simulink model "AutoLIB"  (R2015a)
settings: Solver=FixedStepDiscrete  StartTime=0.0  StopTime=10  FixedStep=0.01  RelTol=1e-3
undefined symbols (not defined in the file or in its folder): sigbuilder_block
settings Model: ModifiedByFormat=Unknown  NumberOfSteps=10  Creator=Unknown  LastModifiedBy=Unknown
settings OptimizationCC: OptimizeModelRefInitCode=on  LifeSpan=1
settings RTWCC: SystemTargetFile=ert.tlc  TemplateMakefile=ert_default_tmf  Description=Embedded Coder
settings CodeAppCC: IgnoreCustomStorageClasses=off
settings ERTTargetCC: ParMdlRefBuildCompliant=on  CompOptLevelCompliant=on  ConcurrentExecutionCompliant=on  ERTFirstTimeCompliant=on  SupportContinuousTime=off  SupportVariableSizeSignals=off  ModelStepFunctionPrototypeControlCompliant=on  CPPClassGenCompliant=on  InlinedParameterPlacement=Hierarchical  ERTCustomFileTemplate=example_file_process.tlc
settings ConfigComp: Description=Design Verifier Custom Configuration Component  DVMaxTestCaseSteps=500  DVTestSuiteOptimization=CombinedObjectives (Nonlinear Extended)

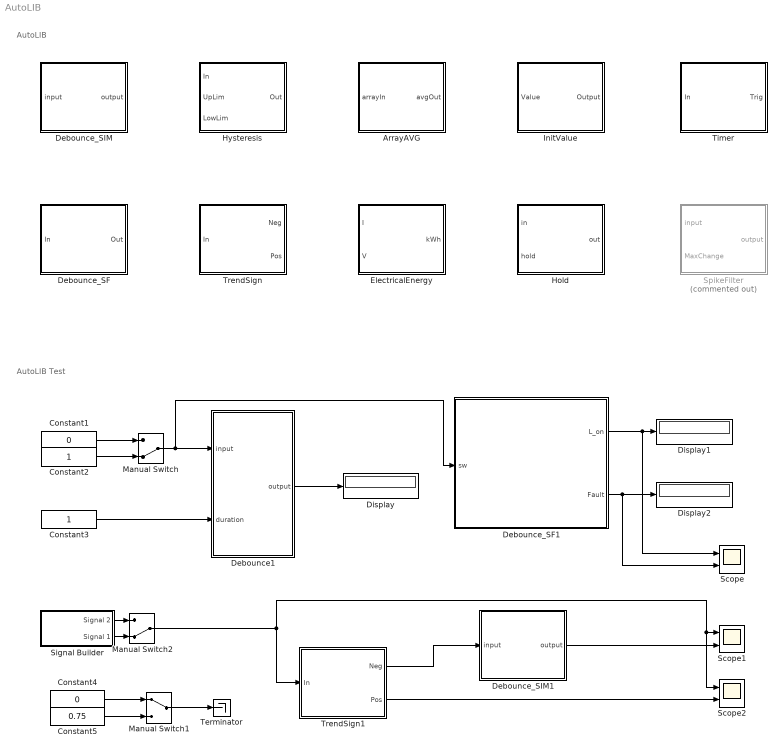
== system AutoLIB ==
  note: AutoLIB
  note: AutoLIB Test
  ArrayAVG : Subsystem  TreatAsAtomicUnit=on
      mask Display:
      | port_label('input',1,'arrIn')
      | port_label('output',1,'avgOut')
      | 
      | 
      | plot([0.30, 0.75],[0.25, 0.25])
      | plot([0.30, 0.30],[0.25, 0.75])
      | 
      | plot([0.55, 0.70],[0.40, 0.40])
      | 
      | color('red');
      | plot([0.30, 0.50],[0.50, 0.50])
      | 
      | color('blue');
      | plot([0.30, 0.50],[0.30, 0.30])
      | 
      | color('green');
      | plot([0.30, 0.50],[0.40, 0.40])
  Constant1 : Constant  Value=0  OutDataTypeStr=boolean
  Constant2 : Constant  OutDataTypeStr=boolean
  Constant3 : Constant  OutDataTypeStr=boolean
  Constant4 : Constant  Value=0  OutDataTypeStr=double
  Constant5 : Constant  Value=0.75  OutDataTypeStr=double
  Debounce1 : Subsystem
  Debounce_SF : Subsystem  TreatAsAtomicUnit=on  mask{Duration=0}
      mask Display:
      | port_label('input',1,'In')
      | port_label('output',1,'Out')
      | 
      | disp(['Debounce: ' num2str(double(Duration)) '\n\n\n\n\n'])
      | 
      | plot([0.30, 0.75],[0.25, 0.25])
      | plot([0.30, 0.30],[0.25, 0.75])
      | 
      | plot([0.30, 0.32],[0.50, 0.50])
      | plot([0.32, 0.32],[0.50, 0.25])
      | plot([0.32, 0.34],[0.25, 0.25])
      | plot([0.34, 0.34],[0.25, 0.50])
      | 
      | plot([0.34, 0.36],[0.50, 0.50])
      | plot([0.36, 0.36],[0.50, 0.25])
      | plot([0.36, 0.38],[0.25, 0.25])
      | plot([0.38, 0.38],[0.25, 0.50])
      | plot([0.38, 0.42],[0.50, 0.50])
      | 
      | color('red');
      | plot([0.42, 0.42],[0.25, 0.50])
      | plot([0.42, 0.52],[0.50, 0.50])
      | plot([0.52, 0.52],[0.50, 0.25])
      | plot([0.52, 0.52],[0.25, 0.25])
  Debounce_SF1 : Stateflow chart  TreatAsAtomicUnit=on
  Debounce_SIM : Subsystem  TreatAsAtomicUnit=on  mask{Duration=3}
      mask prompts: Duration "Debounce Duration"
      mask help: The bouncing action can produce transient signals that do not represent a true change of state, Debounce block avoids these bouncing state.
      mask Display:
      | port_label('input',1,'In')
      | port_label('output',1,'Out')
      | 
      | disp(['Debounce: ' num2str(double(Duration)) '\n\n\n\n\n'])
      | 
      | plot([0.30, 0.75],[0.25, 0.25])
      | plot([0.30, 0.30],[0.25, 0.75])
      | 
      | plot([0.30, 0.32],[0.50, 0.50])
      | plot([0.32, 0.32],[0.50, 0.25])
      | plot([0.32, 0.34],[0.25, 0.25])
      | plot([0.34, 0.34],[0.25, 0.50])
      | 
      | plot([0.34, 0.36],[0.50, 0.50])
      | plot([0.36, 0.36],[0.50, 0.25])
      | plot([0.36, 0.38],[0.25, 0.25])
      | plot([0.38, 0.38],[0.25, 0.50])
      | plot([0.38, 0.42],[0.50, 0.50])
      | 
      | color('red');
      | plot([0.42, 0.42],[0.25, 0.50])
      | plot([0.42, 0.52],[0.50, 0.50])
      | plot([0.52, 0.52],[0.50, 0.25])
      | plot([0.52, 0.52],[0.25, 0.25])
  Debounce_SIM1 : Subsystem  mask{Duration=2}
      mask prompts: Duration "Debounce Duration"
      mask help: The bouncing action can produce transient signals that do not represent a true change of state, Debounce block avoids these bouncing state.
      mask Display:
      | port_label('input',1,'In')
      | port_label('output',1,'Out')
      | 
      | disp(['Debounce: ' num2str(double(Duration)) '\n\n\n\n\n'])
      | 
      | plot([0.30, 0.75],[0.25, 0.25])
      | plot([0.30, 0.30],[0.25, 0.75])
      | 
      | plot([0.30, 0.32],[0.50, 0.50])
      | plot([0.32, 0.32],[0.50, 0.25])
      | plot([0.32, 0.34],[0.25, 0.25])
      | plot([0.34, 0.34],[0.25, 0.50])
      | 
      | plot([0.34, 0.36],[0.50, 0.50])
      | plot([0.36, 0.36],[0.50, 0.25])
      | plot([0.36, 0.38],[0.25, 0.25])
      | plot([0.38, 0.38],[0.25, 0.50])
      | plot([0.38, 0.42],[0.50, 0.50])
      | 
      | color('red');
      | plot([0.42, 0.42],[0.25, 0.50])
      | plot([0.42, 0.52],[0.50, 0.50])
      | plot([0.52, 0.52],[0.50, 0.25])
      | plot([0.52, 0.52],[0.25, 0.25])
  Display : Display
  Display1 : Display
  Display2 : Display
  ElectricalEnergy : Subsystem  TreatAsAtomicUnit=on  mask{SampleTime=0}
      mask Display: plot([10 20 30 40], [10 20 10 15])
  Hold : Subsystem  TreatAsAtomicUnit=on  mask{StepTime=0.01}
      mask prompts: StepTime "Sample Time"
      mask help: Output is fixed at TRUE for HOLD TIME after falling edge of Input.
      mask Display:
      | port_label('input',1,'In')
      | port_label('input',2,'Hold')
      | port_label('output',1,'Out')
      | 
      | plot([0.30, 0.75],[0.25, 0.25])
      | plot([0.30, 0.30],[0.25, 0.75])
      | plot([0.30, 0.60],[0.50, 0.50])
      | plot([0.60, 0.60],[0.50, 0.25])
  Hysteresis : Subsystem  TreatAsAtomicUnit=on
      mask Display:
      | plot([10 20 30 40], [10 20 10 15])
      | color('red');
      | plot([10 40], [17 17])
      | plot([10 40], [13 13])
  InitValue : Subsystem  TreatAsAtomicUnit=on  mask{InitValue=3, SampleTime=-1}
      mask Display:
      | disp(['Initial value: ' num2str(double(InitValue)) '\n\n\n\n'])
      | 
      | plot([0.30, 0.75],[0.25, 0.25])
      | plot([0.30, 0.30],[0.25, 0.75])
      | 
      | plot([0.30, 0.32],[0.50, 0.50])
      | plot([0.34, 0.36],[0.50, 0.50])
      | plot([0.38, 0.40],[0.50, 0.50])
      | plot([0.42, 0.44],[0.50, 0.50])
      | plot([0.46, 0.48],[0.50, 0.50])
      | 
      | plot([0.50, 0.60],[0.50, 0.50])
      | plot([0.60, 0.60],[0.50, 0.25])
  Manual Switch : ManualSwitch  CurrentSetting=0
  Manual Switch1 : ManualSwitch
  Manual Switch2 : ManualSwitch  CurrentSetting=0
  Scope : Scope  NumInputPorts=2
      settings: YMin=0~0  YMax=1~1
  Scope1 : Scope  NumInputPorts=2
      settings: YMin=-0.01~-1  YMax=-0.0092~1
  Scope2 : Scope  NumInputPorts=2
      settings: YMin=-0.01~-1  YMax=-0.0092~1  SaveName=ScopeData2
  Signal Builder : Subsystem  Tag=STV Subsys  LoadFcn=sigbuilder_block('load');  StartFcn=sigbuilder_block('start');  StopFcn=sigbuilder_block('stop');  ClipboardFcn=sigbuilder_block('clipboard');  mask(Sigbuilder block){}
      mask help: Simulink:masks:SigbuilderBlock_MD
      mask init:
      | if ~strcmp(get_param(bdroot(gcbh),'SimulationStatus'),'stopped') tuvar = sigbuilder_block('maskInit'); end
      settings: CopyFcn=sigbuilder_block('copy');  DeleteFcn=sigbuilder_block('delete');  ModelCloseFcn=sigbuilder_block('modelClose');  PreSaveFcn=sigbuilder_block('preSave');  PauseFcn=sigbuilder_block('pause');  ContinueFcn=sigbuilder_block('continue');  NameChangeFcn=sigbuilder_block('namechange');  OpenFcn=sigbuilder_block('open',[437.6 199.2 550.4 400 ]);  CloseFcn=sigbuilder_block('close');
      mask Display: plot(0, 0, 100, 100,[2, 2, 32, 32, 2], [68, 8, 8, 68, 68],[32, 2], [38, 38], [32, 19, 2],[53, 60, 44], [32, 17, 17, 2],[16, 16, 31, 31]);txt = getActiveGroup(gcbh);text(2, 100, txt,'verticalAlignment', 'top');
  SpikeFilter : Subsystem  Commented=on
  Terminator : Terminator
  Timer : Subsystem  TreatAsAtomicUnit=on  mask{Limit=3}
      mask Display:
      | disp(['Timer Target: ' num2str(double(Limit)) '\n\n\n\n'])
      | 
      | 
      | plot([0.30, 0.75],[0.30, 0.30])
      | plot([0.30, 0.30],[0.30, 0.70])
      | plot([0.30, 0.45],[0.30, 0.60])
      | 
      | 
      | color('red');
      | plot([0.45, 0.75],[0.60, 0.60])
  TrendSign : Subsystem  TreatAsAtomicUnit=on
      settings: MinAlgLoopOccurrences=on
      mask Display: fprintf('d/dt');
  TrendSign1 : Subsystem
      mask Display: fprintf('d/dt');
  wires:
  Manual Switch/1 -> Debounce1/1(input), Debounce_SF1/1(sw)
  Constant3/1 -> Debounce1/2(duration)
  Constant1/1 -> Manual Switch/1
  Debounce_SF1/1(L_on) -> Scope/1, Display1/1
  Debounce_SF1/2(Fault) -> Scope/2, Display2/1
  Debounce1/1(output) -> Display/1
  Constant2/1 -> Manual Switch/2
  Manual Switch1/1 -> Terminator/1
  Constant4/1 -> Manual Switch1/1
  Constant5/1 -> Manual Switch1/2
  Signal Builder/1(Signal 2) -> Manual Switch2/1
  Signal Builder/2(Signal 1) -> Manual Switch2/2
  Manual Switch2/1 -> TrendSign1/1(In), Scope2/1, Scope1/1
  Debounce_SIM1/1(output) -> Scope1/2
  TrendSign1/1(Neg) -> Debounce_SIM1/1(input)
  TrendSign1/2(Pos) -> Scope2/2

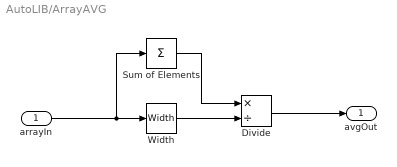
== system AutoLIB/ArrayAVG ==
  arrayIn : Inport
  Divide : Product  Inputs=*/
  Sum of Elements : Sum  Inputs=+
  Width : Width
  avgOut : Outport
  wires:
  Sum of Elements/1 -> Divide/1
  Width/1 -> Divide/2
  arrayIn/1 -> Width/1, Sum of Elements/1
  Divide/1 -> avgOut/1

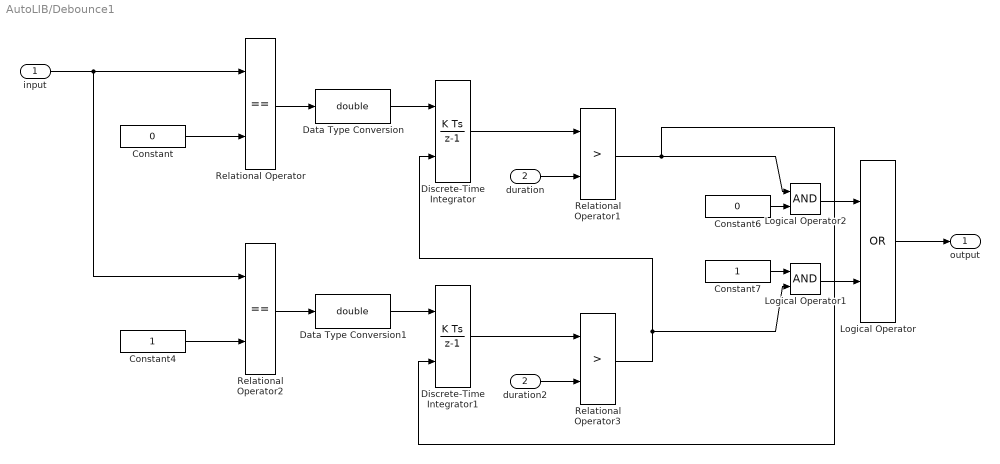
== system AutoLIB/Debounce1 ==
  input : Inport
  duration : Inport  Port=2
  Constant : Constant  Value=0  OutDataTypeStr=boolean
  Constant4 : Constant  OutDataTypeStr=boolean
  Constant6 : Constant  Value=0  OutDataTypeStr=boolean
  Constant7 : Constant  OutDataTypeStr=boolean
  Data Type Conversion : DataTypeConversion  OutDataTypeStr=double
  Data Type Conversion1 : DataTypeConversion  OutDataTypeStr=double
  Discrete-Time Integrator : DiscreteIntegrator  ExternalReset=rising  InitialConditionSetting=State (most efficient)  SampleTime=0.01
  Discrete-Time Integrator1 : DiscreteIntegrator  ExternalReset=rising  InitialConditionSetting=State (most efficient)  SampleTime=0.01
  Logical Operator : Logic  Operator=OR  AllPortsSameDT=off  OutDataTypeStr=boolean
  Logical Operator1 : Logic  AllPortsSameDT=off  OutDataTypeStr=boolean
  Logical Operator2 : Logic  AllPortsSameDT=off  OutDataTypeStr=boolean
  Relational Operator : RelationalOperator  Operator===  OutDataTypeStr=boolean
  Relational Operator1 : RelationalOperator  Operator=>  OutDataTypeStr=boolean
  Relational Operator2 : RelationalOperator  Operator===  OutDataTypeStr=boolean
  Relational Operator3 : RelationalOperator  Operator=>  OutDataTypeStr=boolean
  duration2 : InportShadow  Port=2
  output : Outport
  wires:
  Constant7/1 -> Logical Operator1/1
  Constant6/1 -> Logical Operator2/2
  Discrete-Time Integrator1/1 -> Relational Operator3/1
  Relational Operator3/1 -> Logical Operator1/2, Discrete-Time Integrator/2
  duration2/1 -> Relational Operator3/2
  input/1 -> Relational Operator/1, Relational Operator2/1
  Relational Operator2/1 -> Data Type Conversion1/1
  Data Type Conversion1/1 -> Discrete-Time Integrator1/1
  Constant4/1 -> Relational Operator2/2
  Data Type Conversion/1 -> Discrete-Time Integrator/1
  Logical Operator/1 -> output/1
  Logical Operator2/1 -> Logical Operator/1
  Logical Operator1/1 -> Logical Operator/2
  Relational Operator1/1 -> Logical Operator2/1, Discrete-Time Integrator1/2
  Relational Operator/1 -> Data Type Conversion/1
  Discrete-Time Integrator/1 -> Relational Operator1/1
  duration/1 -> Relational Operator1/2
  Constant/1 -> Relational Operator/2

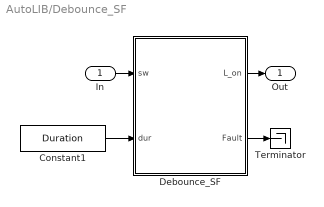
== system AutoLIB/Debounce_SF ==
  In : Inport
  Constant1 : Constant  Value=Duration  SampleTime=-1
  Debounce_SF : Stateflow chart  TreatAsAtomicUnit=on
  Terminator : Terminator
  Out : Outport
  wires:
  In/1 -> Debounce_SF/1(sw)
  Debounce_SF/1(L_on) -> Out/1
  Debounce_SF/2(Fault) -> Terminator/1
  Constant1/1 -> Debounce_SF/2(dur)

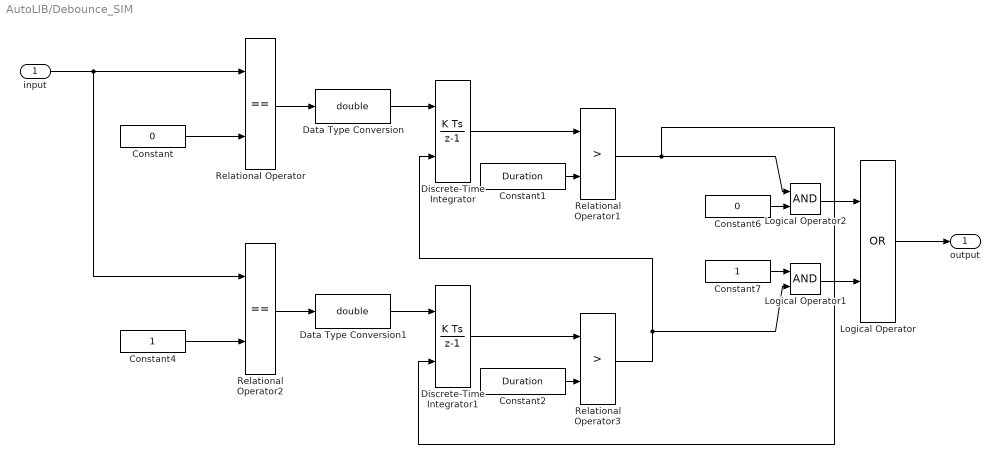
== system AutoLIB/Debounce_SIM ==
  input : Inport
  Constant : Constant  Value=0  OutDataTypeStr=boolean
  Constant1 : Constant  Value=Duration  SampleTime=-1
  Constant2 : Constant  Value=Duration  SampleTime=-1
  Constant4 : Constant  OutDataTypeStr=boolean
  Constant6 : Constant  Value=0  OutDataTypeStr=boolean
  Constant7 : Constant  OutDataTypeStr=boolean
  Data Type Conversion : DataTypeConversion  OutDataTypeStr=double
  Data Type Conversion1 : DataTypeConversion  OutDataTypeStr=double
  Discrete-Time Integrator : DiscreteIntegrator  ExternalReset=rising  InitialConditionSetting=State (most efficient)  SampleTime=0.01
  Discrete-Time Integrator1 : DiscreteIntegrator  ExternalReset=rising  InitialConditionSetting=State (most efficient)  SampleTime=0.01
  Logical Operator : Logic  Operator=OR  AllPortsSameDT=off  OutDataTypeStr=boolean
  Logical Operator1 : Logic  AllPortsSameDT=off  OutDataTypeStr=boolean
  Logical Operator2 : Logic  AllPortsSameDT=off  OutDataTypeStr=boolean
  Relational Operator : RelationalOperator  Operator===  OutDataTypeStr=boolean
  Relational Operator1 : RelationalOperator  Operator=>  OutDataTypeStr=boolean
  Relational Operator2 : RelationalOperator  Operator===  OutDataTypeStr=boolean
  Relational Operator3 : RelationalOperator  Operator=>  OutDataTypeStr=boolean
  output : Outport
  wires:
  Constant/1 -> Relational Operator/2
  Constant1/1 -> Relational Operator1/2
  Discrete-Time Integrator/1 -> Relational Operator1/1
  Relational Operator/1 -> Data Type Conversion/1
  Relational Operator1/1 -> Discrete-Time Integrator1/2, Logical Operator2/1
  Logical Operator1/1 -> Logical Operator/2
  Logical Operator2/1 -> Logical Operator/1
  Logical Operator/1 -> output/1
  Data Type Conversion/1 -> Discrete-Time Integrator/1
  Constant4/1 -> Relational Operator2/2
  Data Type Conversion1/1 -> Discrete-Time Integrator1/1
  Relational Operator2/1 -> Data Type Conversion1/1
  input/1 -> Relational Operator2/1, Relational Operator/1
  Relational Operator3/1 -> Discrete-Time Integrator/2, Logical Operator1/2
  Discrete-Time Integrator1/1 -> Relational Operator3/1
  Constant6/1 -> Logical Operator2/2
  Constant7/1 -> Logical Operator1/1
  Constant2/1 -> Relational Operator3/2

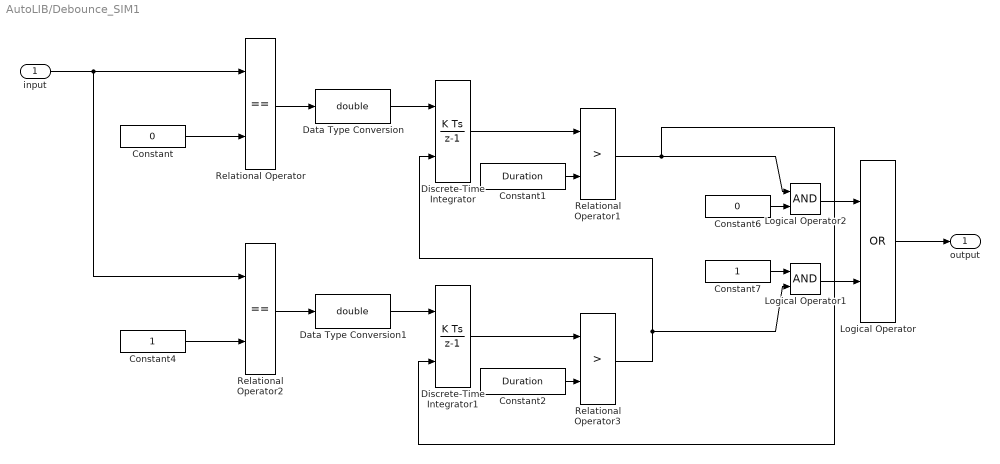
== system AutoLIB/Debounce_SIM1 ==
  input : Inport
  Constant : Constant  Value=0  OutDataTypeStr=boolean
  Constant1 : Constant  Value=Duration  SampleTime=-1
  Constant2 : Constant  Value=Duration  SampleTime=-1
  Constant4 : Constant  OutDataTypeStr=boolean
  Constant6 : Constant  Value=0  OutDataTypeStr=boolean
  Constant7 : Constant  OutDataTypeStr=boolean
  Data Type Conversion : DataTypeConversion  OutDataTypeStr=double
  Data Type Conversion1 : DataTypeConversion  OutDataTypeStr=double
  Discrete-Time Integrator : DiscreteIntegrator  ExternalReset=rising  InitialConditionSetting=State (most efficient)  SampleTime=0.01
  Discrete-Time Integrator1 : DiscreteIntegrator  ExternalReset=rising  InitialConditionSetting=State (most efficient)  SampleTime=0.01
  Logical Operator : Logic  Operator=OR  AllPortsSameDT=off  OutDataTypeStr=boolean
  Logical Operator1 : Logic  AllPortsSameDT=off  OutDataTypeStr=boolean
  Logical Operator2 : Logic  AllPortsSameDT=off  OutDataTypeStr=boolean
  Relational Operator : RelationalOperator  Operator===  OutDataTypeStr=boolean
  Relational Operator1 : RelationalOperator  Operator=>  OutDataTypeStr=boolean
  Relational Operator2 : RelationalOperator  Operator===  OutDataTypeStr=boolean
  Relational Operator3 : RelationalOperator  Operator=>  OutDataTypeStr=boolean
  output : Outport
  wires:
  Constant2/1 -> Relational Operator3/2
  Constant7/1 -> Logical Operator1/1
  Constant6/1 -> Logical Operator2/2
  Discrete-Time Integrator1/1 -> Relational Operator3/1
  Relational Operator3/1 -> Logical Operator1/2, Discrete-Time Integrator/2
  input/1 -> Relational Operator/1, Relational Operator2/1
  Relational Operator2/1 -> Data Type Conversion1/1
  Data Type Conversion1/1 -> Discrete-Time Integrator1/1
  Constant4/1 -> Relational Operator2/2
  Data Type Conversion/1 -> Discrete-Time Integrator/1
  Logical Operator/1 -> output/1
  Logical Operator2/1 -> Logical Operator/1
  Logical Operator1/1 -> Logical Operator/2
  Relational Operator1/1 -> Logical Operator2/1, Discrete-Time Integrator1/2
  Relational Operator/1 -> Data Type Conversion/1
  Discrete-Time Integrator/1 -> Relational Operator1/1
  Constant1/1 -> Relational Operator1/2
  Constant/1 -> Relational Operator/2

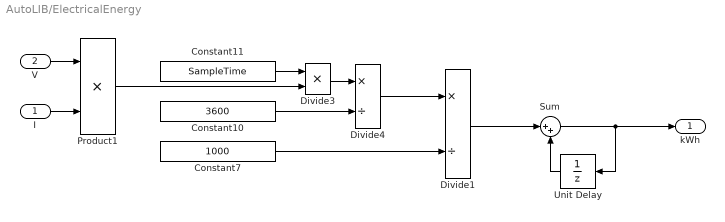
== system AutoLIB/ElectricalEnergy ==
  I : Inport
  V : Inport  Port=2
  Constant10 : Constant  Value=3600  SampleTime=-1
  Constant11 : Constant  Value=SampleTime  SampleTime=-1
  Constant7 : Constant  Value=1000  SampleTime=-1
  Divide1 : Product  Inputs=*/
  Divide3 : Product  Inputs=**
  Divide4 : Product  Inputs=*/
  Product1 : Product  Inputs=**
  Sum : Sum  Inputs=|++
  Unit Delay : UnitDelay  SampleTime=-1
  kWh : Outport
  wires:
  Product1/1 -> Divide3/2
  I/1 -> Product1/2
  Constant7/1 -> Divide1/2
  Constant11/1 -> Divide3/1
  Divide4/1 -> Divide1/1
  Divide3/1 -> Divide4/1
  V/1 -> Product1/1
  Unit Delay/1 -> Sum/2
  Sum/1 -> Unit Delay/1, kWh/1
  Divide1/1 -> Sum/1
  Constant10/1 -> Divide4/2

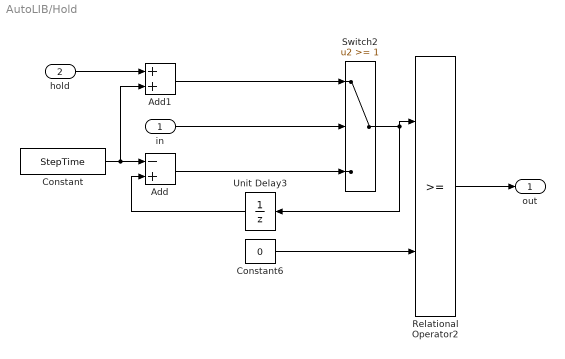
== system AutoLIB/Hold ==
  in : Inport
  hold : Inport  Port=2
  Add : Sum  Inputs=-+
  Add1 : Sum
  Constant : Constant  Value=StepTime  SampleTime=-1
  Constant6 : Constant  Value=0  OutDataTypeStr=double  SampleTime=StepTime
  Relational Operator2 : RelationalOperator  SampleTime=StepTime  InputSameDT=on
  Switch2 : Switch  Threshold=1  SampleTime=StepTime  SaturateOnIntegerOverflow=on  InputSameDT=on
  Unit Delay3 : UnitDelay  SampleTime=StepTime
  out : Outport
  wires:
  Switch2/1 -> Relational Operator2/1, Unit Delay3/1
  in/1 -> Switch2/2
  Relational Operator2/1 -> out/1
  Constant6/1 -> Relational Operator2/2
  Constant/1 -> Add1/2, Add/1
  Add1/1 -> Switch2/1
  Add/1 -> Switch2/3
  Unit Delay3/1 -> Add/2
  hold/1 -> Add1/1

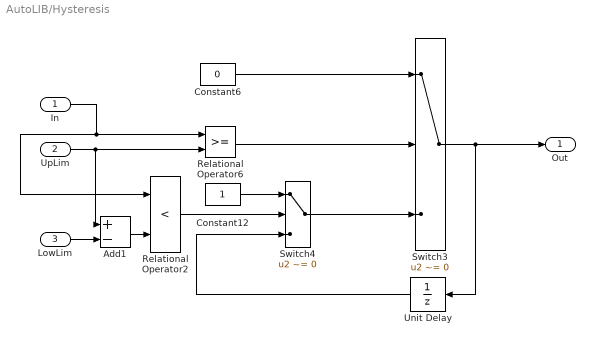
== system AutoLIB/Hysteresis ==
  In : Inport
  UpLim : Inport  Port=2
  LowLim : Inport  Port=3
  Add1 : Sum  Inputs=+-
  Constant12 : Constant  OutDataTypeStr=boolean  SampleTime=-1
  Constant6 : Constant  Value=0  OutDataTypeStr=boolean  SampleTime=-1
  Relational Operator2 : RelationalOperator  Operator=<  OutDataTypeStr=boolean
  Relational Operator6 : RelationalOperator  OutDataTypeStr=boolean
  Switch3 : Switch  Criteria=u2 ~= 0
  Switch4 : Switch  Criteria=u2 ~= 0
  Unit Delay : UnitDelay  SampleTime=-1
  Out : Outport
  wires:
  Constant6/1 -> Switch3/1
  UpLim/1 -> Add1/1, Relational Operator6/2
  In/1 -> Relational Operator2/1, Relational Operator6/1
  Switch3/1 -> Unit Delay/1, Out/1
  Switch4/1 -> Switch3/3
  Relational Operator2/1 -> Switch4/2
  LowLim/1 -> Add1/2
  Relational Operator6/1 -> Switch3/2
  Unit Delay/1 -> Switch4/3
  Constant12/1 -> Switch4/1
  Add1/1 -> Relational Operator2/2

== system AutoLIB/InitValue ==
  Value : Inport
  Constant : Constant  Value=InitValue  SampleTime=-1
  Switch : Switch  Criteria=u2 ~= 0  Threshold=0.5
  Output : Outport
  wires:
  Constant/1 -> Switch/3
  Switch/1 -> Output/1
  Value/1 -> Switch/2, Switch/1

== system AutoLIB/Signal Builder ==
  Demux : Demux  Tag=STV Demux  Outputs=2
  FromWs : FromWorkspace  Tag=STV FromWs  VariableName=tuvar  SampleTime=0
      SigBuilderData=|
      | common.afterFinalStr = 'Extrapolate'
      | common.sampleTime = 0
      | dataSet.timeRange = [0 10]
      | dataSet.name = 'Group 1'
      | sbobj.Groups.Name = 'Group 1'
      | sbobj.Groups.Signals(1).Name = 'Signal 2'
      | sbobj.Groups.Signals(1).XData = [0 1 1 2 2 3 3 4 4 5 5 6 6 7 7 8 8 9 9 10]
      | sbobj.Groups.Signals(1).YData = [0 2 0 2 0 2 0 2 0 2 0 2 0 2 0 2 0 2 0 2]
      | sbobj.Groups.Signals(2).Name = 'Signal 1'
      | sbobj.Groups.Signals(2).XData = [0 2 2 3.04 3.04 6.01 6.01 10]
      | sbobj.Groups.Signals(2).YData = [0 0 1 1 0.54 -0.46 0 1]
  Signal 2 : Outport  Tag=STV Outport
  Signal 1 : Outport  Tag=STV Outport  Port=2
  wires:
  FromWs/1 -> Demux/1
  Demux/1 -> Signal 2/1
  Demux/2 -> Signal 1/1

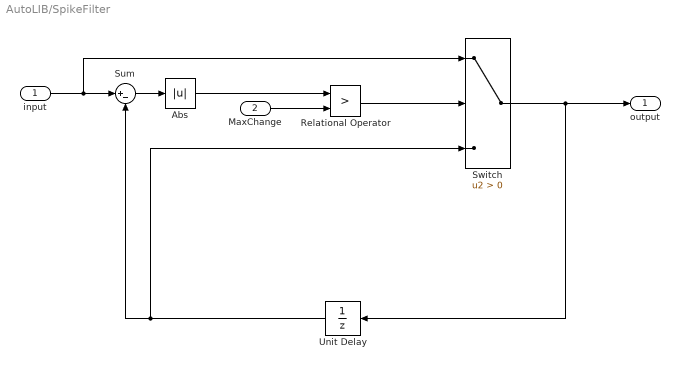
== system AutoLIB/SpikeFilter ==
  input : Inport
  MaxChange : Inport  Port=2
  Abs : Abs
  Relational Operator : RelationalOperator  Operator=>  OutDataTypeStr=boolean
  Sum : Sum  Inputs=|+-
  Switch : Switch  Criteria=u2 > Threshold
  Unit Delay : UnitDelay  SampleTime=-1
  output : Outport
  wires:
  input/1 -> Sum/1, Switch/1
  Unit Delay/1 -> Switch/3, Sum/2
  Sum/1 -> Abs/1
  MaxChange/1 -> Relational Operator/2
  Relational Operator/1 -> Switch/2
  Switch/1 -> output/1, Unit Delay/1
  Abs/1 -> Relational Operator/1

== system AutoLIB/Timer ==
  In : Inport
  Constant : Constant  Value=Limit  SampleTime=-1
  Timer : Stateflow chart  TreatAsAtomicUnit=on
  Trig : Outport
  wires:
  Constant/1 -> Timer/2(limit)
  Timer/1(out) -> Trig/1
  In/1 -> Timer/1(in)

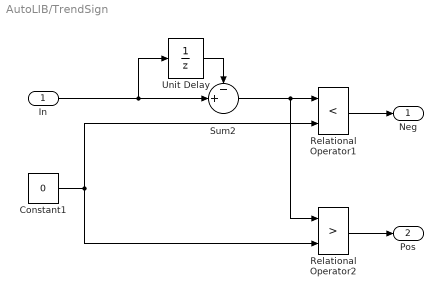
== system AutoLIB/TrendSign ==
  In : Inport
  Constant1 : Constant  Value=0  OutDataTypeStr=int8  SampleTime=-1
  Relational Operator1 : RelationalOperator  Operator=<  OutDataTypeStr=boolean
  Relational Operator2 : RelationalOperator  Operator=>  OutDataTypeStr=boolean
  Sum2 : Sum  Inputs=-+|  OutDataTypeStr=Inherit: Inherit via back propagation  SaturateOnIntegerOverflow=on
  Unit Delay : UnitDelay  SampleTime=-1
  Neg : Outport
  Pos : Outport  Port=2
  wires:
  Constant1/1 -> Relational Operator2/2, Relational Operator1/2
  Sum2/1 -> Relational Operator1/1, Relational Operator2/1
  Unit Delay/1 -> Sum2/1
  In/1 -> Unit Delay/1, Sum2/2
  Relational Operator1/1 -> Neg/1
  Relational Operator2/1 -> Pos/1

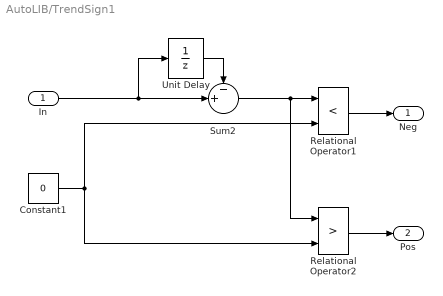
== system AutoLIB/TrendSign1 ==
  In : Inport
  Constant1 : Constant  Value=0  OutDataTypeStr=int8  SampleTime=-1
  Relational Operator1 : RelationalOperator  Operator=<  OutDataTypeStr=boolean
  Relational Operator2 : RelationalOperator  Operator=>  OutDataTypeStr=boolean
  Sum2 : Sum  Inputs=-+|  SaturateOnIntegerOverflow=on
  Unit Delay : UnitDelay  SampleTime=-1
  Neg : Outport
  Pos : Outport  Port=2
  wires:
  Relational Operator2/1 -> Pos/1
  Relational Operator1/1 -> Neg/1
  In/1 -> Sum2/2, Unit Delay/1
  Unit Delay/1 -> Sum2/1
  Sum2/1 -> Relational Operator2/1, Relational Operator1/1
  Constant1/1 -> Relational Operator1/2, Relational Operator2/2

== stateflow chart AutoLIB/Debounce_SF1 ==
  state Off
    en: L_on = 0;
    state Normal
      en: Fault = 0;
    state Fault
      en: Fault = 1;
    Fault -> Normal : after(1,sec)
    (default) -> Normal
  state Debounce
    state On
      en: L_on = 1;
    state Off
      en: L_on = 0;
    Debounce.Off -> Debounce.On [order 2] : [sw>0]
    Debounce.On -> Debounce.Off [order 1] : [sw<1]
  state On
    en: L_on = 1;
  (default) -> Off
  Normal -> Debounce.On : [sw>0]
  Debounce.Off -> Fault [order 1] : after(0.1,sec)
  Debounce -> Fault : after(0.3,sec)
  Debounce.On -> On [order 2] : after(0.1,sec)
  (junction 23) -> Debounce.Off : after(1,sec)
  On -> (junction 23) : [sw<1]
  data: sw input; L_on output; Fault output

== stateflow chart AutoLIB/Timer/Timer ==
  state Timer
    state out
      on after(limit,sec):
      out = 1;
    state in
      en: out=0;
    (default) -> in
    in -> out : [in == 1]
    out -> in : [in == 0]
  (default) -> Timer
  data: in input; out output; limit input

== stateflow chart AutoLIB/Debounce_SF/Debounce_SF ==
  state Off
    en: L_on = 0;
    state Normal
      en: Fault = 0;
    state Fault
      en: Fault = 1;
    Fault -> Normal : after(dur*10,sec)
    (default) -> Normal
  state Debounce
    state On
      en: L_on = 1;
    state Off
      en: L_on = 0;
    Debounce.Off -> Debounce.On [order 2] : [sw>0]
    Debounce.On -> Debounce.Off [order 1] : [sw<1]
  state On
    en: L_on = 1;
  (default) -> Off
  Normal -> Debounce.On : [sw>0]
  Debounce.Off -> Fault [order 1] : after(dur,sec)
  Debounce -> Fault : after(dur,sec)
  Debounce.On -> On [order 2] : after(dur, sec)
  (junction 23) -> Debounce.Off : after(dur, sec)
  On -> (junction 23) : [sw<1]
  data: sw input; L_on output; Fault output; dur input
